simulink subsystem "GenericApplyModulation"  (R2024a)
settings: Solver=VariableStepAuto  StartTime=0.0  StopTime=10.0  RelTol=1e-3
settings Model: Creator=dfurodet  LastModifiedBy=dfurodet

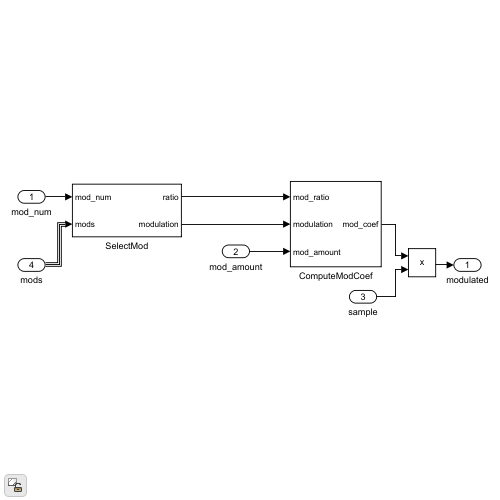
[thumbnail: Simulink's stored preview of the top-level diagram]
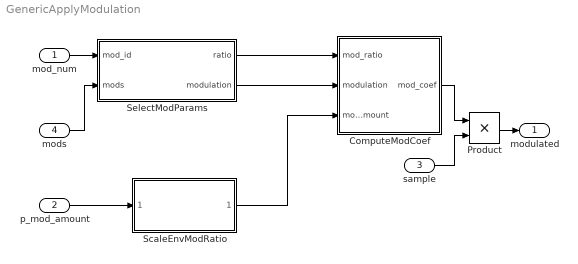
== system GenericApplyModulation ==
  mod_num : Inport  OutDataTypeStr=uint8
  p_mod_amount : Inport  Port=2
  sample : Inport  Port=3
  mods : Inport  Port=4
  ComputeModCoef : Subsystem
  Product : Product
  ScaleEnvModRatio : Subsystem  ReferencedSubsystem=ScaleU8Param
  SelectModParams : MATLAB Function  TreatAsAtomicUnit=on
  modulated : Outport
  wires:
  ComputeModCoef/1(mod_coef) -> Product/1
  sample/1 -> Product/2
  Product/1 -> modulated/1
  p_mod_amount/1 -> ScaleEnvModRatio/1
  ScaleEnvModRatio/1 -> ComputeModCoef/3(mod_amount)
  mod_num/1 -> SelectModParams/1(mod_id)
  mods/1 -> SelectModParams/2(mods)
  SelectModParams/1(ratio) -> ComputeModCoef/1(mod_ratio)
  SelectModParams/2(modulation) -> ComputeModCoef/2(modulation)

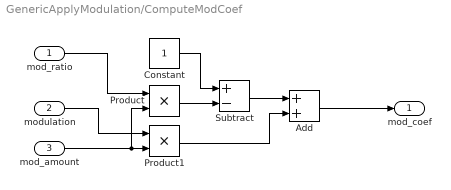
== system GenericApplyModulation/ComputeModCoef ==
  mod_ratio : Inport
  modulation : Inport  Port=2
  mod_amount : Inport  Port=3
  Add : Sum
  Constant : Constant  OutDataTypeStr=single
  Product : Product
  Product1 : Product
  Subtract : Sum  Inputs=+-
  mod_coef : Outport
  wires:
  Add/1 -> mod_coef/1
  Constant/1 -> Subtract/1
  modulation/1 -> Product1/1
  mod_ratio/1 -> Product/1
  Product1/1 -> Add/2
  mod_amount/1 -> Product/2, Product1/2
  Product/1 -> Subtract/2
  Subtract/1 -> Add/1

== matlab function GenericApplyModulation/SelectModParams ==
  data: mod_id input; mods input; ratio output; modulation output
function [ratio, modulation] = fcn(mod_id, mods)
ratio = mods(2 * mod_id + 1);
modulation = mods(2 * mod_id + 2);
